simulink model "momentum_dump_test_rev2"  (R2016b)
settings: Solver=VariableStepAuto  StartTime=0.0  StopTime=2400  MinStep=0.001  RelTol=1e-3
values from neighbouring files (symbols this model uses):
  fsw_params = init_fsw_params()    [momentum_unload_test_init.m]
undefined symbols (not defined in the file): sim_params
libraries: simulink x3, dynamics_lib x1, environment_lib x1, pd_control_lib x1, aerolibutil x1, RW_assembly_simple_lib x1, command_processing x1
settings Model: Creator=evich  LastModifiedBy=evich

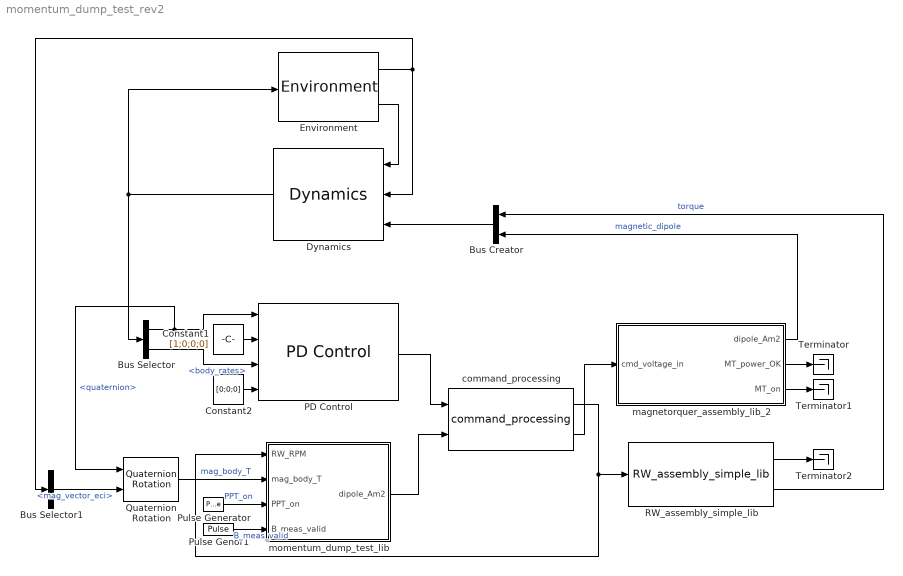
== system momentum_dump_test_rev2 ==
  Bus Creator : BusCreator  Inputs=2
  Bus Selector : BusSelector  OutputSignals=quaternion,body_rates
  Bus Selector1 : BusSelector  OutputSignals=mag_vector_eci
  Constant1 : Constant  Value=[1;0;0;0]
  Constant2 : Constant  Value=[0;0;0]
  Dynamics : dynamics_lib/Dynamics
  Environment : environment_lib/Environment
  PD Control : pd_control_lib/PD Control
  Pulse Generator : DiscretePulseGenerator  PulseType=Time based  Period=fsw_params.actuators.ppt.sync_pulse  PulseWidth=fsw_params.actuators.ppt.t_charge_pct
  Pulse Genor1 : DiscretePulseGenerator  PulseType=Time based  Period=10  PulseWidth=sim_params.sensors.magnetometer.valid_pct
  Quaternion Rotation : aerolibutil/Quaternion Rotation
  RW_assembly_simple_lib : RW_assembly_simple_lib/RW_assembly_simple_lib  natural_frequency=sim_params.actuators.reaction_wheel.natural_freq  damping_ratio=sim_params.actuators.reaction_wheel.damping  max_rate=sim_params.actuators.reaction_wheel.rate_limit
  Terminator : Terminator
  Terminator1 : Terminator
  Terminator2 : Terminator
  command_processing : command_processing/command_processing
  magnetorquer_assembly_lib_2 : Subsystem
  momentum_dump_test_lib : Subsystem
  wires:
  Dynamics/1 -> Bus Selector/1, Environment/1
  Environment/2 -> Dynamics/1
  Environment/1 -> Dynamics/2, Bus Selector1/1
  Bus Creator/1 -> Dynamics/3
  RW_assembly_simple_lib/2 -> Bus Creator/1  "torque"
  magnetorquer_assembly_lib_2/1(dipole_Am2) -> Bus Creator/2  "magnetic_dipole"
  Bus Selector/1 -> Quaternion Rotation/1, PD Control/1  "<quaternion>"
  Bus Selector/2 -> PD Control/3  "<body_rates>"
  command_processing/1 -> momentum_dump_test_lib/1(RW_RPM), RW_assembly_simple_lib/1
  command_processing/2 -> magnetorquer_assembly_lib_2/1(cmd_voltage_in)
  PD Control/1 -> command_processing/1
  momentum_dump_test_lib/1(dipole_Am2) -> command_processing/2
  Pulse Generator/1 -> momentum_dump_test_lib/3(PPT_on)  "PPT_on"
  Pulse Genor1/1 -> momentum_dump_test_lib/4(B_meas_valid)  "B_meas_valid"
  Constant1/1 -> PD Control/2
  Constant2/1 -> PD Control/4
  magnetorquer_assembly_lib_2/2(MT_power_OK) -> Terminator/1
  magnetorquer_assembly_lib_2/3(MT_on) -> Terminator1/1
  RW_assembly_simple_lib/1 -> Terminator2/1
  Bus Selector1/1 -> Quaternion Rotation/2  "<mag_vector_eci>"
  Quaternion Rotation/1 -> momentum_dump_test_lib/2(mag_body_T)  "mag_body_T"

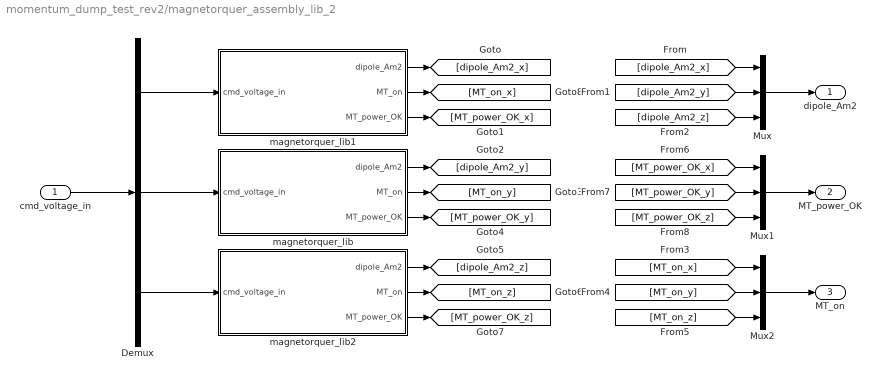
== system momentum_dump_test_rev2/magnetorquer_assembly_lib_2 ==
  cmd_voltage_in : Inport
  Demux : Demux  Outputs=3
  Mux : Mux  Inputs=3
  Mux1 : Mux  Inputs=3
  Mux2 : Mux  Inputs=3
  magnetorquer_lib : Subsystem  mask{voltage_to_dipole=0.25*sim_params.actuators.magnetorquer.max_dipole_y, upperbound=sim_params.actuators.magnetorquer.max_dipole_y, lowerbound=-sim_params.actuators.magnetorquer.max_dipole_y}
      mask prompts: voltage_to_dipole "Simulink:blkprm_prompts:GainGain"; upperbound "Simulink:masks:UpperBound_MP"; lowerbound "Simulink:masks:LowerBound_MP"
      mask TypeOptions voltage_to_dipole: Gain/Gain
      mask TypeOptions upperbound:
      | Check
      | Static Range/max
      mask TypeOptions lowerbound:
      | Check
      | Static Range/min
  magnetorquer_lib1 : Subsystem  mask{voltage_to_dipole=0.25*sim_params.actuators.magnetorquer.max_dipole_x, upperbound=sim_params.actuators.magnetorquer.max_dipole_x, lowerbound=-sim_params.actuators.magnetorquer.max_dipole_x}
      mask prompts: voltage_to_dipole "Simulink:blkprm_prompts:GainGain"; upperbound "Simulink:masks:UpperBound_MP"; lowerbound "Simulink:masks:LowerBound_MP"
      mask TypeOptions voltage_to_dipole: Gain/Gain
      mask TypeOptions upperbound:
      | Check
      | Static Range/max
      mask TypeOptions lowerbound:
      | Check
      | Static Range/min
  magnetorquer_lib2 : Subsystem  mask{voltage_to_dipole=0.25*sim_params.actuators.magnetorquer.max_dipole_z, upperbound=sim_params.actuators.magnetorquer.max_dipole_z, lowerbound=-sim_params.actuators.magnetorquer.max_dipole_z}
      mask prompts: voltage_to_dipole "Simulink:blkprm_prompts:GainGain"; upperbound "Simulink:masks:UpperBound_MP"; lowerbound "Simulink:masks:LowerBound_MP"
      mask TypeOptions voltage_to_dipole: Gain/Gain
      mask TypeOptions upperbound:
      | Check
      | Static Range/max
      mask TypeOptions lowerbound:
      | Check
      | Static Range/min
  dipole_Am2 : Outport
  MT_power_OK : Outport  Port=2
  MT_on : Outport  Port=3
  wires:
  cmd_voltage_in/1 -> Demux/1
  Demux/3 -> magnetorquer_lib2/1(cmd_voltage_in)
  Demux/1 -> magnetorquer_lib1/1(cmd_voltage_in)
  Demux/2 -> magnetorquer_lib/1(cmd_voltage_in)
  magnetorquer_lib1/1(dipole_Am2) -> [dipole_Am2_x]
  magnetorquer_lib2/3(MT_power_OK) -> [MT_power_OK_z]
  magnetorquer_lib2/2(MT_on) -> [MT_on_z]
  magnetorquer_lib2/1(dipole_Am2) -> [dipole_Am2_z]
  magnetorquer_lib/3(MT_power_OK) -> [MT_power_OK_y]
  magnetorquer_lib/2(MT_on) -> [MT_on_y]
  magnetorquer_lib/1(dipole_Am2) -> [dipole_Am2_y]
  magnetorquer_lib1/3(MT_power_OK) -> [MT_power_OK_x]
  magnetorquer_lib1/2(MT_on) -> [MT_on_x]
  Mux/1 -> dipole_Am2/1
  Mux1/1 -> MT_power_OK/1
  Mux2/1 -> MT_on/1
  [dipole_Am2_x] -> Mux/1
  [dipole_Am2_y] -> Mux/2
  [dipole_Am2_z] -> Mux/3
  [MT_on_x] -> Mux2/1
  [MT_on_y] -> Mux2/2
  [MT_on_z] -> Mux2/3
  [MT_power_OK_x] -> Mux1/1
  [MT_power_OK_y] -> Mux1/2
  [MT_power_OK_z] -> Mux1/3

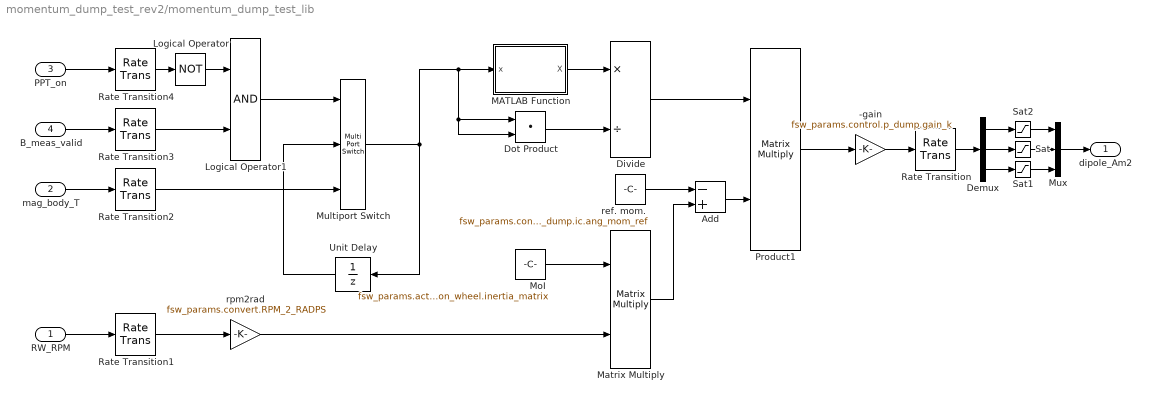
== system momentum_dump_test_rev2/momentum_dump_test_lib ==
  RW_RPM : Inport
  mag_body_T : Inport  Port=2
  PPT_on : Inport  Port=3
  B_meas_valid : Inport  Port=4
  -gain : Gain  Gain=fsw_params.control.p_dump.gain_k
  Add : Sum  Inputs=-+
  Demux : Demux  Outputs=3
  Divide : Product  Inputs=*/
  Dot Product : DotProduct  InputSameDT=on  OutDataTypeStr=Inherit: Inherit via internal rule
  Logical Operator : Logic  Operator=NOT  AllPortsSameDT=off  OutDataTypeStr=boolean
  Logical Operator1 : Logic  AllPortsSameDT=off  OutDataTypeStr=boolean
  MATLAB Function : MATLAB Function  TreatAsAtomicUnit=on
  Matrix Multiply : Product  Inputs=**  Multiplication=Matrix(*)
  MoI : Constant  Value=fsw_params.actuators.reaction_wheel.inertia_matrix
  Multiport Switch : MultiPortSwitch  DataPortOrder=Zero-based contiguous  Inputs=2
  Mux : Mux  Inputs=3
  Product1 : Product  Inputs=**  Multiplication=Matrix(*)
  Rate Transition : RateTransition  X0=fsw_params.control.p_dump.ic.rt_dipole_Am2
  Rate Transition1 : RateTransition  X0=fsw_params.control.p_dump.ic.rt_w_body_radps  OutPortSampleTime=fsw_params.control.p_dump.sample_time_s
  Rate Transition2 : RateTransition  X0=fsw_params.control.p_dump.ic.rt_mag_body_T  OutPortSampleTime=fsw_params.control.p_dump.sample_time_s
  Rate Transition3 : RateTransition  X0=fsw_params.control.p_dump.ic.rt_B_meas_valid  OutPortSampleTime=fsw_params.control.p_dump.sample_time_s
  Rate Transition4 : RateTransition  X0=fsw_params.control.p_dump.ic.rt_PPT_on  OutPortSampleTime=fsw_params.control.p_dump.sample_time_s
  Sat : Saturate  UpperLimit=fsw_params.actuators.magnetorquer.max_dipole_y  LowerLimit=-fsw_params.actuators.magnetorquer.max_dipole_y
  Sat1 : Saturate  UpperLimit=fsw_params.actuators.magnetorquer.max_dipole_z  LowerLimit=-fsw_params.actuators.magnetorquer.max_dipole_z
  Sat2 : Saturate  UpperLimit=fsw_params.actuators.magnetorquer.max_dipole_x  LowerLimit=-fsw_params.actuators.magnetorquer.max_dipole_x
  Unit Delay : UnitDelay  InitialCondition=fsw_params.control.p_dump.ic.delay  SampleTime=-1
  ref. mom. : Constant  Value=fsw_params.control.p_dump.ic.ang_mom_ref
  rpm2rad : Gain  Gain=fsw_params.convert.RPM_2_RADPS
  dipole_Am2 : Outport
  wires:
  Dot Product/1 -> Divide/2
  ref. mom./1 -> Add/1
  Matrix Multiply/1 -> Add/2
  MATLAB Function/1(X) -> Divide/1
  MoI/1 -> Matrix Multiply/1
  Multiport Switch/1 -> MATLAB Function/1(x), Dot Product/2, Dot Product/1, Unit Delay/1
  rpm2rad/1 -> Matrix Multiply/2
  Add/1 -> Product1/2
  Divide/1 -> Product1/1
  Product1/1 -> -gain/1
  Logical Operator1/1 -> Multiport Switch/1
  Logical Operator/1 -> Logical Operator1/1
  Rate Transition3/1 -> Logical Operator1/2
  Rate Transition4/1 -> Logical Operator/1
  Rate Transition2/1 -> Multiport Switch/3
  Unit Delay/1 -> Multiport Switch/2
  PPT_on/1 -> Rate Transition4/1
  B_meas_valid/1 -> Rate Transition3/1
  mag_body_T/1 -> Rate Transition2/1
  RW_RPM/1 -> Rate Transition1/1
  Rate Transition1/1 -> rpm2rad/1
  Rate Transition/1 -> Demux/1
  Demux/2 -> Sat/1
  Demux/1 -> Sat2/1
  Demux/3 -> Sat1/1
  Sat1/1 -> Mux/3
  Sat/1 -> Mux/2
  Sat2/1 -> Mux/1
  Mux/1 -> dipole_Am2/1
  -gain/1 -> Rate Transition/1

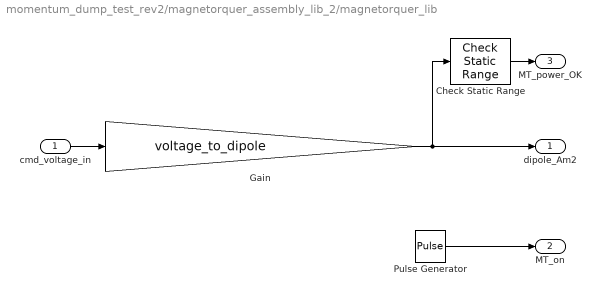
== system momentum_dump_test_rev2/magnetorquer_assembly_lib_2/magnetorquer_lib ==
  cmd_voltage_in : Inport
  Check Static Range : simulink/Model Verification/Check  Static Range  Description=lowerbound <= u <= upperbound  max=upperbound  max_included=on  min=lowerbound  min_included=on  enabled=on  stopWhenAssertionFail=off  export=on  icon=graphic
  Gain : Gain  Gain=voltage_to_dipole
  Pulse Generator : DiscretePulseGenerator  PulseType=Time based  Period=1  PulseWidth=fsw_params.actuators.magnetorquer.actuation_time_pct
  dipole_Am2 : Outport
  MT_on : Outport  Port=2
  MT_power_OK : Outport  Port=3
  wires:
  cmd_voltage_in/1 -> Gain/1
  Gain/1 -> Check Static Range/1, dipole_Am2/1
  Pulse Generator/1 -> MT_on/1
  Check Static Range/1 -> MT_power_OK/1

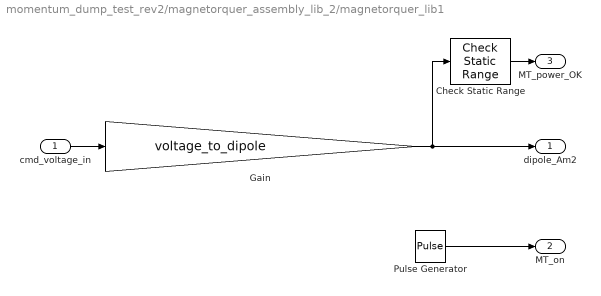
== system momentum_dump_test_rev2/magnetorquer_assembly_lib_2/magnetorquer_lib1 ==
  cmd_voltage_in : Inport
  Check Static Range : simulink/Model Verification/Check  Static Range  Description=lowerbound <= u <= upperbound  max=upperbound  max_included=on  min=lowerbound  min_included=on  enabled=on  stopWhenAssertionFail=off  export=on  icon=graphic
  Gain : Gain  Gain=voltage_to_dipole
  Pulse Generator : DiscretePulseGenerator  PulseType=Time based  Period=1  PulseWidth=fsw_params.actuators.magnetorquer.actuation_time_pct
  dipole_Am2 : Outport
  MT_on : Outport  Port=2
  MT_power_OK : Outport  Port=3
  wires:
  cmd_voltage_in/1 -> Gain/1
  Gain/1 -> Check Static Range/1, dipole_Am2/1
  Pulse Generator/1 -> MT_on/1
  Check Static Range/1 -> MT_power_OK/1

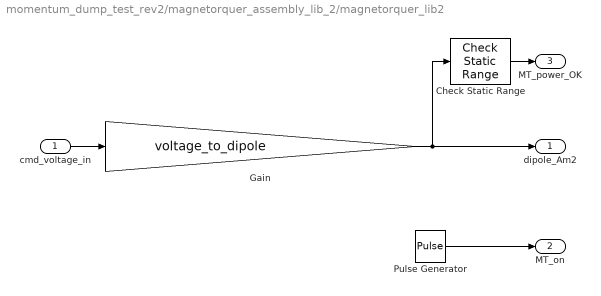
== system momentum_dump_test_rev2/magnetorquer_assembly_lib_2/magnetorquer_lib2 ==
  cmd_voltage_in : Inport
  Check Static Range : simulink/Model Verification/Check  Static Range  Description=lowerbound <= u <= upperbound  max=upperbound  max_included=on  min=lowerbound  min_included=on  enabled=on  stopWhenAssertionFail=off  export=on  icon=graphic
  Gain : Gain  Gain=voltage_to_dipole
  Pulse Generator : DiscretePulseGenerator  PulseType=Time based  Period=1  PulseWidth=fsw_params.actuators.magnetorquer.actuation_time_pct
  dipole_Am2 : Outport
  MT_on : Outport  Port=2
  MT_power_OK : Outport  Port=3
  wires:
  cmd_voltage_in/1 -> Gain/1
  Gain/1 -> Check Static Range/1, dipole_Am2/1
  Pulse Generator/1 -> MT_on/1
  Check Static Range/1 -> MT_power_OK/1

== matlab function momentum_dump_test_rev2/momentum_dump_test_lib/MATLAB Function ==
  data: x input; X output
function X   = skew( x )
% UW HuskySat-1, ADCS Subsystem
% Last Update: E. Hansen 12.8.2017

%Transforms a vector into a skew symmetric matrix (Levi-Civita)
%--------------------------------------------------------------------------

X = [0 -x(3) x(2);x(3) 0 -x(1);-x(2) x(1) 0];
